simulink model "Question3"  (R2023b)
settings: Solver=VariableStepAuto  StartTime=0.0  StopTime=20.0  RelTol=1e-3
values from neighbouring files (symbols this model uses):
  den1 = cell2mat(HY3_N1_D.denominator)    [ThreeDiskOscillator.m]
  den2 = cell2mat(HY3_N2_D.denominator)    [ThreeDiskOscillator.m]
  num_HU2_N1_D = cell2mat(HU2_N1_D.numerator)    [ThreeDiskOscillator.m]
  num_HY1_N1_D = cell2mat(HY1_N1_D.numerator)    [ThreeDiskOscillator.m]
  num_HY2_N1_D = cell2mat(HY2_N1_D.numerator)    [ThreeDiskOscillator.m]
  num_HY2_N2_D = cell2mat(HY2_N2_D.numerator)    [ThreeDiskOscillator.m]
  num_HY3_N1_D = cell2mat(HY3_N1_D.numerator)    [ThreeDiskOscillator.m]
  num_HY3_N2_D = cell2mat(HY3_N2_D.numerator)    [ThreeDiskOscillator.m]
undefined symbols (not defined in the file or in its folder): den
settings Model: Creator=andre  LastModifiedBy=andre

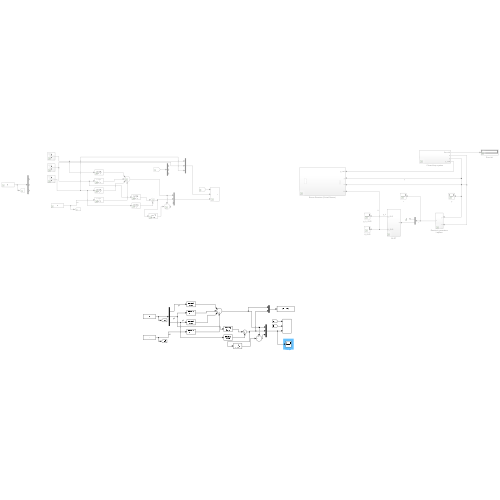
[thumbnail: Simulink's stored preview of the top-level diagram]
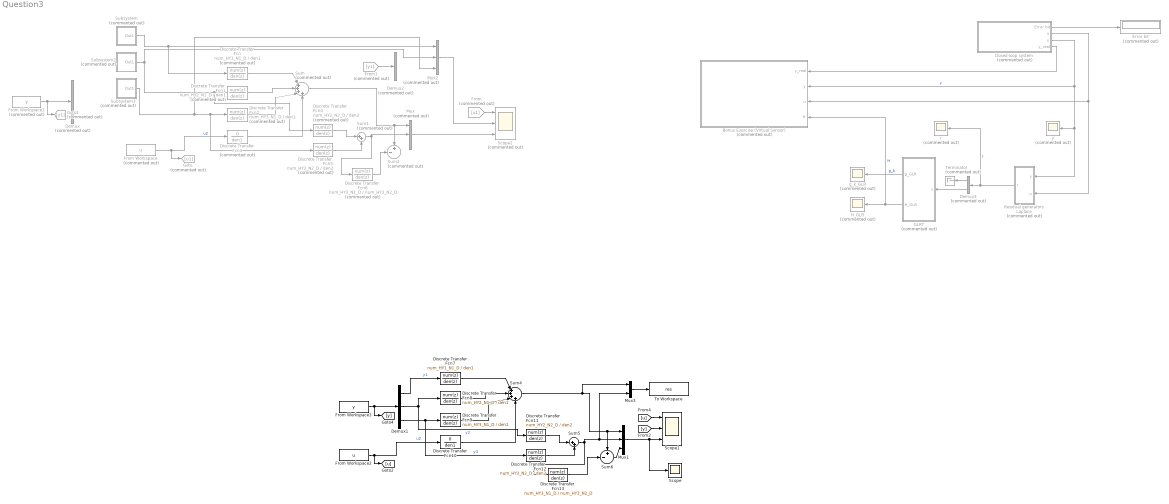
== system Question3 ==
  " H_GLR" : Scope  Commented=on
  " g_k_GLR" : Scope  Commented=on
  " r" : Scope  Commented=on
  " y" : Scope  Commented=on
  Bonus Exercise (Virtual Sensor) : Subsystem  Commented=on
  Closed-loop system : Subsystem  Commented=on
  Demux : Demux  Commented=on  Outputs=3
  Demux1 : Demux  Outputs=3
  Demux2 : Demux  Commented=on  Outputs=3
  Demux3 : Demux  Commented=on  Outputs=2
  Discrete Transfer Fcn : DiscreteTransferFcn  Commented=on  Numerator=num_HY1_N1_D  Denominator=den1
  Discrete Transfer Fcn1 : DiscreteTransferFcn  Commented=on  Numerator=num_HY2_N1_D  Denominator=den1
  Discrete Transfer Fcn10 : DiscreteTransferFcn  Numerator=0  Denominator=den1
  Discrete Transfer Fcn11 : DiscreteTransferFcn  Numerator=num_HY2_N2_D  Denominator=den2
  Discrete Transfer Fcn12 : DiscreteTransferFcn  Numerator=num_HY3_N2_D  Denominator=den2
  Discrete Transfer Fcn13 : DiscreteTransferFcn  Numerator=num_HY3_N1_D  Denominator=num_HY3_N2_D
  Discrete Transfer Fcn2 : DiscreteTransferFcn  Commented=on  Numerator=num_HY3_N1_D  Denominator=den1
  Discrete Transfer Fcn3 : DiscreteTransferFcn  Commented=on  Numerator=0  Denominator=den1
  Discrete Transfer Fcn4 : DiscreteTransferFcn  Commented=on  Numerator=num_HY2_N2_D  Denominator=den2
  Discrete Transfer Fcn5 : DiscreteTransferFcn  Commented=on  Numerator=num_HY3_N2_D  Denominator=den2
  Discrete Transfer Fcn6 : DiscreteTransferFcn  Commented=on  Numerator=num_HY3_N1_D  Denominator=num_HY3_N2_D
  Discrete Transfer Fcn7 : DiscreteTransferFcn  Numerator=num_HY1_N1_D  Denominator=den1
  Discrete Transfer Fcn8 : DiscreteTransferFcn  Numerator=num_HY2_N1_D  Denominator=den1
  Discrete Transfer Fcn9 : DiscreteTransferFcn  Numerator=num_HY3_N1_D  Denominator=den1
  "Error bit " : Display  Commented=on
  From : From  Commented=on  GotoTag=u1
  From Workspace : FromWorkspace  Commented=on  VariableName=u
  From Workspace1 : FromWorkspace  Commented=on  VariableName=y  SampleTime=0.004
  From Workspace2 : FromWorkspace  VariableName=u
  From Workspace3 : FromWorkspace  VariableName=y  SampleTime=0.004
  From1 : From  Commented=on  GotoTag=y1
  GLRT : Subsystem  Commented=on
  Goto : Goto  Commented=on  GotoTag=u1
  Goto1 : Goto  Commented=on  GotoTag=y1
  Mux : Mux  Commented=on  Inputs=3
  Mux1 : Mux  Inputs=3
  Mux2 : Mux  Commented=on  Inputs=3
  Mux3 : Mux  Inputs=2
  Residual generators Laplace : Subsystem  Commented=on
  Scope : Scope
  Scope1 : Scope  NumInputPorts=3
  Scope2 : Scope  Commented=on  NumInputPorts=3
  Subsystem : Subsystem  Commented=on
  Subsystem2 : Subsystem  Commented=on
  Subsystem3 : Subsystem  Commented=on
  Sum : Sum  Commented=on  Inputs=|++++
  Sum1 : Sum  Commented=on  Inputs=|++
  Sum2 : Sum  Commented=on  Inputs=+-|
  Sum4 : Sum  Inputs=|++++
  Sum5 : Sum  Inputs=|++
  Sum6 : Sum  Inputs=+-|
  Terminator : Terminator  Commented=on
  To Workspace : ToWorkspace  VariableName=res  SaveFormat=Structure With Time  SampleTime=-1
  wires:
  Mux/1 -> Scope2/3
  Sum1/1 -> Mux/2, Discrete Transfer Fcn6/1
  Discrete Transfer Fcn4/1 -> Sum1/1
  From Workspace/1 -> Goto/1, Discrete Transfer Fcn3/1  "u2"
  Discrete Transfer Fcn5/1 -> Sum1/2
  Discrete Transfer Fcn3/1 -> Sum/4
  Discrete Transfer Fcn1/1 -> Sum/2
  Discrete Transfer Fcn2/1 -> Sum/3
  From Workspace1/1 -> Goto1/1, Demux/1
  From/1 -> Scope2/1
  Discrete Transfer Fcn6/1 -> Sum2/2
  Sum/1 -> Sum2/1, Mux/1
  Discrete Transfer Fcn/1 -> Sum/1
  Discrete Transfer Fcn8/1 -> Sum4/2
  Discrete Transfer Fcn13/1 -> Sum6/2
  Discrete Transfer Fcn10/1 -> Sum4/4
  Demux1/3 -> Discrete Transfer Fcn12/1, Discrete Transfer Fcn9/1  "y3"
  Discrete Transfer Fcn7/1 -> Sum4/1
  [y] -> Scope1/2
  From Workspace3/1 -> [y], Demux1/1
  Discrete Transfer Fcn9/1 -> Sum4/3
  Demux1/1 -> Discrete Transfer Fcn7/1  "y1"
  Demux1/2 -> Discrete Transfer Fcn8/1, Discrete Transfer Fcn11/1  "y2"
  Discrete Transfer Fcn12/1 -> Sum5/2
  Sum5/1 -> Mux3/2, Mux1/2, Discrete Transfer Fcn13/1
  Discrete Transfer Fcn11/1 -> Sum5/1
  Mux1/1 -> Scope/1, Scope1/3
  Sum6/1 -> Mux1/3
  From Workspace2/1 -> Discrete Transfer Fcn10/1, [u]  "u2"
  [u] -> Scope1/1
  From1/1 -> Demux2/1
  Mux2/1 -> Scope2/2
  Subsystem/1(Out1) -> Discrete Transfer Fcn/1, Mux2/1
  Subsystem2/1(Out1) -> Discrete Transfer Fcn4/1, Discrete Transfer Fcn1/1, Mux2/2
  Subsystem3/1(Out1) -> Mux2/3, Discrete Transfer Fcn5/1, Discrete Transfer Fcn2/1
  Mux3/1 -> To Workspace/1
  Closed-loop system/1(Error bit) -> "Error bit "/1
  Demux3/2 -> GLRT/1(z)
  GLRT/1(g_GLR) -> " g_k_GLR"/1  "g_k"
  Closed-loop system/2(u) -> Residual generators Laplace/2(u), Bonus Exercise (Virtual Sensor)/3(u)
  Residual generators Laplace/1(r) -> Demux3/1, " r"/1  "r"
  Demux3/1 -> Terminator/1
  Closed-loop system/4(y_real) -> Bonus Exercise (Virtual Sensor)/1(y_real)
  Closed-loop system/3(y) -> Residual generators Laplace/1(y), " y"/1, Bonus Exercise (Virtual Sensor)/2(y)  "y"
  GLRT/2(H_GLR) -> Bonus Exercise (Virtual Sensor)/4(H), " H_GLR"/1  "H"
  Sum4/1 -> Mux3/1, Mux1/1, Sum6/1

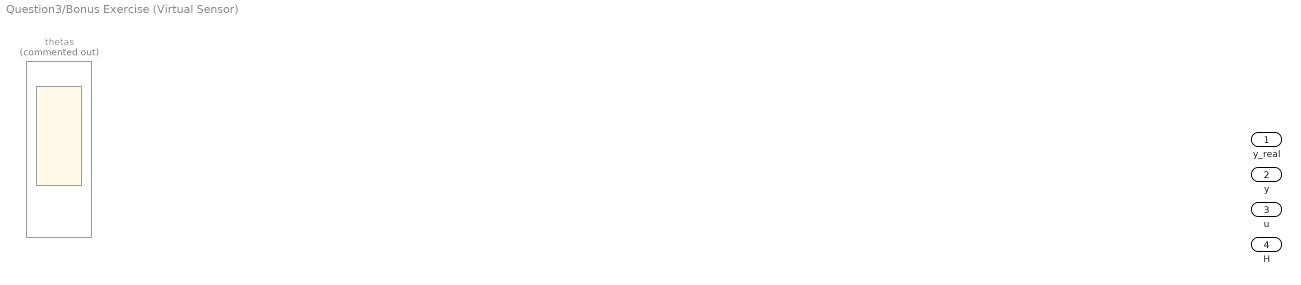
== system Question3/Bonus Exercise (Virtual Sensor) ==
  y_real : Inport
  y : Inport  Port=2
  u : Inport  Port=3
  H : Inport  Port=4
  thetas : Scope  Commented=on  NumInputPorts=3

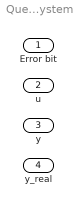
== system Question3/Closed-loop system ==
  Error bit : Outport  VectorParamsAs1DForOutWhenUnconnected=off
  u : Outport  Port=2  VectorParamsAs1DForOutWhenUnconnected=off
  y : Outport  Port=3  VectorParamsAs1DForOutWhenUnconnected=off
  y_real : Outport  Port=4  VectorParamsAs1DForOutWhenUnconnected=off

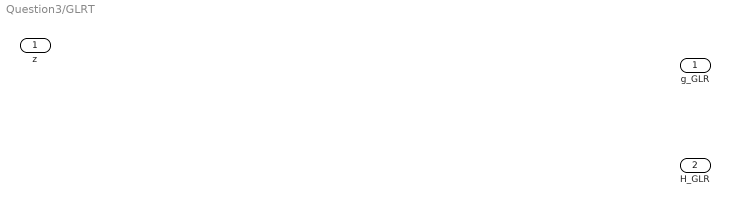
== system Question3/GLRT ==
  z : Inport
  g_GLR : Outport  VectorParamsAs1DForOutWhenUnconnected=off
  H_GLR : Outport  Port=2  VectorParamsAs1DForOutWhenUnconnected=off

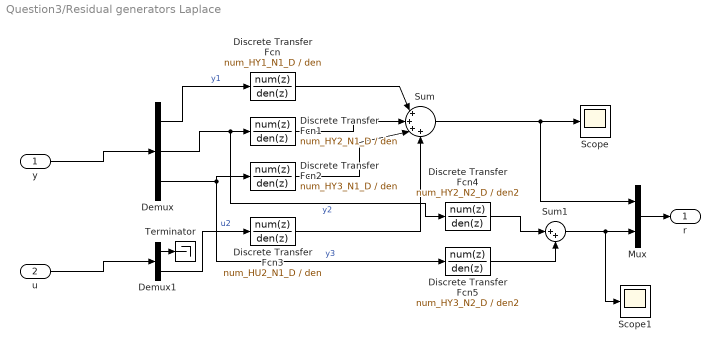
== system Question3/Residual generators Laplace ==
  y : Inport
  u : Inport  Port=2
  Demux : Demux  Outputs=3
  Demux1 : Demux  Outputs=2
  Discrete Transfer Fcn : DiscreteTransferFcn  Numerator=num_HY1_N1_D  Denominator=den
  Discrete Transfer Fcn1 : DiscreteTransferFcn  Numerator=num_HY2_N1_D  Denominator=den
  Discrete Transfer Fcn2 : DiscreteTransferFcn  Numerator=num_HY3_N1_D  Denominator=den
  Discrete Transfer Fcn3 : DiscreteTransferFcn  Numerator=num_HU2_N1_D  Denominator=den
  Discrete Transfer Fcn4 : DiscreteTransferFcn  Numerator=num_HY2_N2_D  Denominator=den2
  Discrete Transfer Fcn5 : DiscreteTransferFcn  Numerator=num_HY3_N2_D  Denominator=den2
  Mux : Mux  Inputs=2
  Scope : Scope
  Scope1 : Scope
  Sum : Sum  Inputs=|++++
  Sum1 : Sum  Inputs=|++
  Terminator : Terminator
  r : Outport  VectorParamsAs1DForOutWhenUnconnected=off
  wires:
  Discrete Transfer Fcn5/1 -> Sum1/2
  Discrete Transfer Fcn/1 -> Sum/1
  Discrete Transfer Fcn1/1 -> Sum/2
  Discrete Transfer Fcn3/1 -> Sum/4
  Demux1/2 -> Discrete Transfer Fcn3/1  "u2"
  Discrete Transfer Fcn2/1 -> Sum/3
  Demux1/1 -> Terminator/1
  Sum1/1 -> Scope1/1, Mux/2
  Mux/1 -> r/1
  Sum/1 -> Scope/1, Mux/1
  Demux/3 -> Discrete Transfer Fcn5/1, Discrete Transfer Fcn2/1  "y3"
  Discrete Transfer Fcn4/1 -> Sum1/1
  Demux/2 -> Discrete Transfer Fcn4/1, Discrete Transfer Fcn1/1  "y2"
  Demux/1 -> Discrete Transfer Fcn/1  "y1"
  y/1 -> Demux/1
  u/1 -> Demux1/1

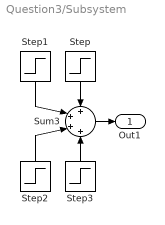
== system Question3/Subsystem ==
  Step : Step  After=1.56  SampleTime=0
  Step1 : Step  Time=5  After=-1.56  SampleTime=0
  Step2 : Step  Time=10  After=1.56  SampleTime=0
  Step3 : Step  Time=15  After=-1.56  SampleTime=0
  Sum3 : Sum  Inputs=++++
  Out1 : Outport
  wires:
  Sum3/1 -> Out1/1
  Step2/1 -> Sum3/3
  Step1/1 -> Sum3/2
  Step3/1 -> Sum3/4
  Step/1 -> Sum3/1

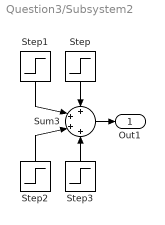
== system Question3/Subsystem2 ==
  Step : Step  After=1.56  SampleTime=0
  Step1 : Step  Time=5  After=-1.56  SampleTime=0
  Step2 : Step  Time=10  After=1.56  SampleTime=0
  Step3 : Step  Time=15  After=-1.56  SampleTime=0
  Sum3 : Sum  Inputs=++++
  Out1 : Outport
  wires:
  Sum3/1 -> Out1/1
  Step2/1 -> Sum3/3
  Step1/1 -> Sum3/2
  Step3/1 -> Sum3/4
  Step/1 -> Sum3/1

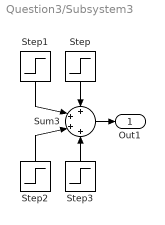
== system Question3/Subsystem3 ==
  Step : Step  After=1.56  SampleTime=0
  Step1 : Step  Time=5  After=-1.56  SampleTime=0
  Step2 : Step  Time=10  After=1.56  SampleTime=0
  Step3 : Step  Time=15  After=-1.40  SampleTime=0
  Sum3 : Sum  Inputs=++++
  Out1 : Outport
  wires:
  Sum3/1 -> Out1/1
  Step2/1 -> Sum3/3
  Step1/1 -> Sum3/2
  Step3/1 -> Sum3/4
  Step/1 -> Sum3/1
